simulink model "robot_data"  (R2015a)
settings: Solver=ode4  StartTime=0.0  StopTime=10  FixedStep=0.01  RelTol=1e-3
settings Model: Creator=LAB425  LastModifiedBy=LAB425

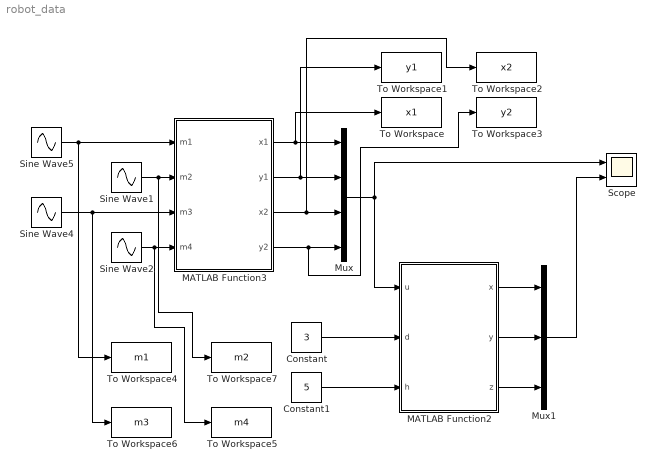
== system robot_data ==
  Constant : Constant  Value=3
  Constant1 : Constant  Value=5
  MATLAB Function2 : MATLAB Function  TreatAsAtomicUnit=on
  MATLAB Function3 : MATLAB Function  TreatAsAtomicUnit=on
  Mux : Mux
  Mux1 : Mux  Inputs=3
  Scope : Scope  NumInputPorts=2
      settings: YMin=-5~-5  YMax=5~5
  Sine Wave1 : Sin  Frequency=2  SampleTime=0
  Sine Wave2 : Sin  Frequency=2  Phase=3.14  SampleTime=0
  Sine Wave4 : Sin  Phase=3.14  SampleTime=0
  Sine Wave5 : Sin  SampleTime=0
  To Workspace : ToWorkspace  VariableName=x1  SaveFormat=Timeseries  SampleTime=-1
  To Workspace1 : ToWorkspace  VariableName=y1  SaveFormat=Timeseries  SampleTime=-1
  To Workspace2 : ToWorkspace  VariableName=x2  SaveFormat=Timeseries  SampleTime=-1
  To Workspace3 : ToWorkspace  VariableName=y2  SaveFormat=Timeseries  SampleTime=-1
  To Workspace4 : ToWorkspace  VariableName=m1  SaveFormat=Timeseries  SampleTime=-1
  To Workspace5 : ToWorkspace  VariableName=m4  SaveFormat=Timeseries  SampleTime=-1
  To Workspace6 : ToWorkspace  VariableName=m3  SaveFormat=Timeseries  SampleTime=-1
  To Workspace7 : ToWorkspace  VariableName=m2  SaveFormat=Timeseries  SampleTime=-1
  wires:
  Constant/1 -> MATLAB Function2/2(d)
  Constant1/1 -> MATLAB Function2/3(h)
  Sine Wave1/1 -> To Workspace7/1, MATLAB Function3/2(m2)
  Sine Wave4/1 -> MATLAB Function3/3(m3), To Workspace6/1
  Sine Wave2/1 -> To Workspace5/1, MATLAB Function3/4(m4)
  MATLAB Function3/2(y1) -> To Workspace1/1, Mux/2
  MATLAB Function3/3(x2) -> To Workspace2/1, Mux/3
  MATLAB Function3/4(y2) -> To Workspace3/1, Mux/4
  Mux/1 -> MATLAB Function2/1(u), Scope/1
  MATLAB Function2/2(y) -> Mux1/2
  MATLAB Function2/1(x) -> Mux1/1
  MATLAB Function2/3(z) -> Mux1/3
  Mux1/1 -> Scope/2
  MATLAB Function3/1(x1) -> To Workspace/1, Mux/1
  Sine Wave5/1 -> MATLAB Function3/1(m1), To Workspace4/1

== matlab function robot_data/MATLAB Function2 ==
  data: x output; u input; y output; z output; d input; h input
function [x,y,z] = Robot(u,d,h)
%按照原有MPC方法，该函数的输入应是对机器人的控制输入量u=（v1,v2,v3,v4）四个电机的当前转速
%考虑传输过程的时延以及噪声误差，在MPC过程利用预测的当前位置作为输入控制量带入
%u=(x1,x2,y1,y2)当前四个丝杆相对固定坐标位置

x1 = u(1);y1 = u(2);x2 = u(3); y2 = u(4);

% T01=[1,0,0,0;0,cos(atan2((x1+x2),d)),-sin(atan2((x1+x2),d)),0;0,sin(atan2((x1+x2),d)),cos(atan2((x1+x2),d)),x1;0,0,0,1];
% T1m=[0,0,1,0;1,0,0,0,;0,1,0,0;0,0,0,1];
% Tmm1=[0,1,0,0;-1,0,0,0;0,0,1,0;0,0,0,1];
% Tm12=[1,0,0,0;0,cos(atan2((y1+y2),d))];
forwardx = sign(x1);forwardy = sign(y1);

X = abs(x1) + abs(x2);
Y = abs(y1) + abs(y2);
L = sqrt(X^2+Y^2);
theta = atan2(L,d);
H = h * sin(theta);
z = -h * cos(theta);
beta = atan2(Y,X);
y = -forwardy * (H * sin(beta) + abs(y2));
x = -forwardx * (H * cos(beta) + abs(x2));

== matlab function robot_data/MATLAB Function3 ==
  data: x1 output; m1 input; y1 output; x2 output; m2 input; m3 input; m4 input; y2 output
function [x1,y1,x2,y2] = Signal(m1,m2,m3,m4)



%m1,m2,m3,m4为四个电机的当前时刻的角度值

%最远距离
D = 2;
% %螺距
% n = 0.02;
% %最大圈数
% ratio = D / n;
v=sqrt(0.01)*randn(4,1);
x1 = m1 * D + v(1);
y1 = m2 * D + v(2);
x2 = m3 * D + v(3);
y2 = m4 * D + v(4);

if x1>=2
    x1=2;
else
    if x1<=-2
        x1=-2;
    end
end
if x2>=2
    x2=2;
else
    if x2<=-2
        x2=-2;
    end
end
if y1>=2
    y1=2;
else
    if y1<=-2
        y1=-2;
    end
end
if y2>=2
    y2=2;
else
    if y2<=-2
        y2=-2;
    end
end
